simulink model "distortion"  (R2014b)
settings: Solver=ode45  StartTime=0.0  StopTime=10.0  RelTol=1e-3
libraries: simulink x1, dspvision x1, dspsnks4 x1
settings Model: Creator=ICLab  LastModifiedBy=ICLab

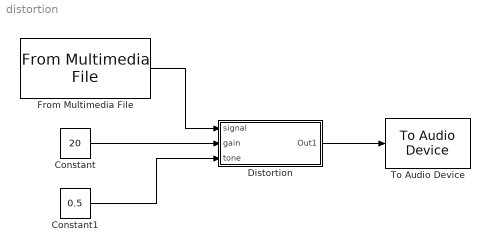
== system distortion ==
  Constant : Constant  Value=20
  Constant1 : Constant  Value=0.5
  Distortion : Subsystem
  From Multimedia File : dspvision/From Multimedia File  inputFilename=C:\Users\ICLab\Desktop\Embedded system\MATLAB_DSP\distortion\harmonyChorus.wav  loop=on  numPlays=inf  outputStreams=Audio only  videoDataType=single  audioDataType=double  inheritSampleTime=on  userDefinedSampleTime=1/30  noAudioOutput=off  isIntensityVideo=off  fourcc=RGB  colorVideoFormat=Separate color signals  outputEOF=off  dataOrg=Column-major  audioFrameSize=2048  computeAudioFrameSize=off  outSamplingMode=Frame based
  To Audio Device : dspsnks4/To Audio Device  deviceName=Default  inheritSampleRate=on  sampleRate=44100  deviceDatatype=Determine from input data type  autoBufferSize=on  bufferSize=4096  queueDuration=1.0  defaultOutputChannelMapping=on  outputChannelMapping=1:2  outputNumUnderrunSamples=off
  wires:
  Constant/1 -> Distortion/2(gain)
  From Multimedia File/1 -> Distortion/1(signal)
  Constant1/1 -> Distortion/3(tone)
  Distortion/1(Out1) -> To Audio Device/1

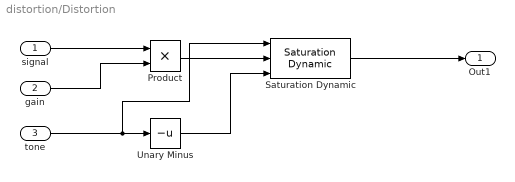
== system distortion/Distortion ==
  signal : Inport
  gain : Inport  Port=2
  tone : Inport  Port=3
  Product : Product
  Saturation Dynamic : simulink/Discontinuities/Saturation Dynamic  OutMin=[]  OutMax=[]  OutDataTypeStr=Inherit: Same as second input  OutDataType=fixdt(1, 16)  OutScaling=2^-10  DoSatur=off
  Unary Minus : UnaryMinus
  Out1 : Outport
  wires:
  signal/1 -> Product/1
  gain/1 -> Product/2
  Product/1 -> Saturation Dynamic/2
  Saturation Dynamic/1 -> Out1/1
  tone/1 -> Saturation Dynamic/1, Unary Minus/1
  Unary Minus/1 -> Saturation Dynamic/3
